simulink model "main_observer_sim1"  (R2015a)
settings: Solver=ode45  StartTime=0.0  StopTime=10  FixedStep=1e-4  MaxStep=1e-3  RelTol=1e-3
values from neighbouring files (symbols this model uses):
  A = sys_rand.A    [main_Observer_states.m]
  C = [0.617255113405149,0,0,-0.448535555941661,0.134230346538703,1.41932930409004;0.283640603624291,0,2.22808153625508,-1.86462753317668,-1.99763494036701,-0.0116516666362024;0.350975702033898,-0.174162030842294,1.44167650824058,-0.392420914284623,1.30288133017051,-0.392171726620127]    [finding_Y.m]    (also in main_Observer_states.m = sys_rand.C)
  Gama = eta*A-X*C    [main_Observer_states.m]    (also in observer.mat = [-0.665415381788 -1.71297839543 -11.0757301234 9.21615917151)
  H = B(:,end)    [main_Observer_states.m]
  Phi = dec2mat(LMISYS,xopt,2)    [main_Observer_states.m]    (also in observer.mat = [2.03974430811 -0.144807404976 -3.64797116197 7.53997403465 )
  theta = theta1+Y*theta2    [main_Observer_states.m]    (also in observer.mat = [-0.848682280391 0.936204937086 2.9983152382 2.21151006385 4)
settings Model: Creator=p4wp4w  LastModifiedBy=p4wp4w

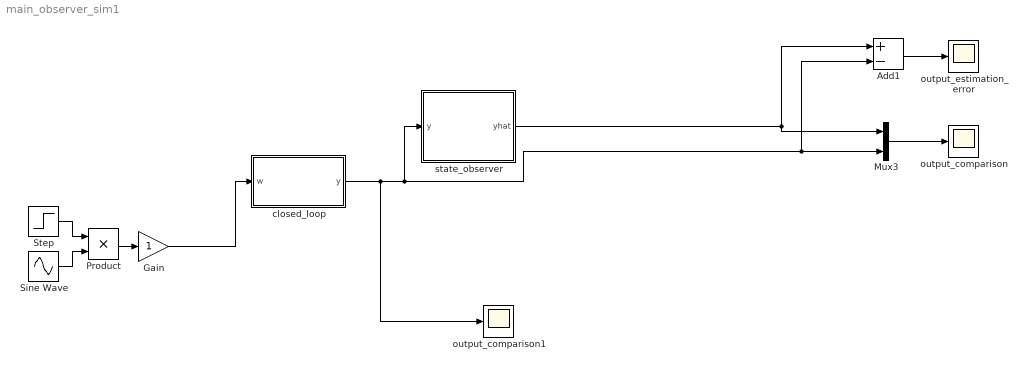
== system main_observer_sim1 ==
  Add1 : Sum  Inputs=+-
  Gain : Gain
  Mux3 : Mux  Inputs=2
  Product : Product
  Sine Wave : Sin  Frequency=10  SampleTime=0
  Step : Step  Before=8  After=0  SampleTime=0
  closed_loop : Subsystem
  output_comparison : Scope
      settings: YMin=-0.00125  YMax=0.003
  output_comparison1 : Scope
      settings: YMin=-0.0024  YMax=-2.1684e-19  SaveName=ScopeData5
  output_estimation_error : Scope
      settings: YMin=-0.0024  YMax=-2.1684e-19  SaveName=errorval
  state_observer : Subsystem
  wires:
  closed_loop/1(y) -> output_comparison1/1, Add1/2, Mux3/2, state_observer/1(y)
  Mux3/1 -> output_comparison/1
  state_observer/1(yhat) -> Mux3/1, Add1/1
  Gain/1 -> closed_loop/1(w)
  Add1/1 -> output_estimation_error/1
  Product/1 -> Gain/1
  Step/1 -> Product/1
  Sine Wave/1 -> Product/2

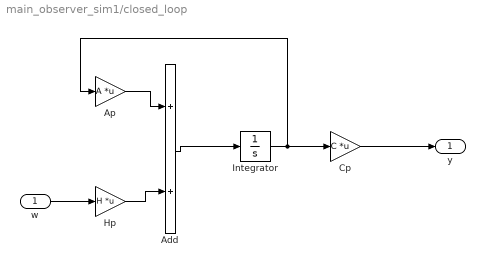
== system main_observer_sim1/closed_loop ==
  w : Inport
  Add : Sum
  Ap : Gain  Gain=A  Multiplication=Matrix(K*u)
  Cp : Gain  Gain=C  Multiplication=Matrix(K*u)
  Hp : Gain  Gain=H  Multiplication=Matrix(K*u)
  Integrator : Integrator
  y : Outport
  wires:
  w/1 -> Hp/1
  Add/1 -> Integrator/1
  Integrator/1 -> Cp/1, Ap/1
  Ap/1 -> Add/1
  Hp/1 -> Add/2
  Cp/1 -> y/1

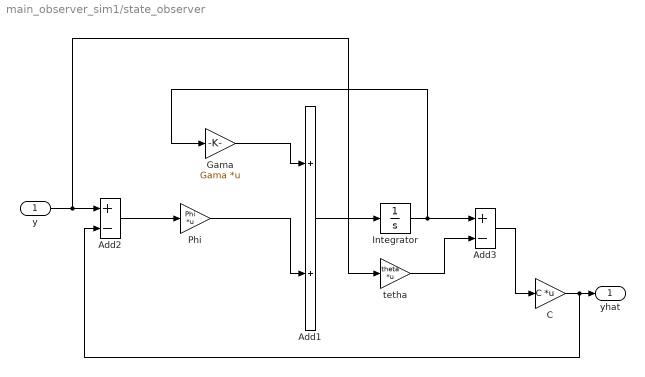
== system main_observer_sim1/state_observer ==
  y : Inport
  Add1 : Sum
  Add2 : Sum  Inputs=+-
  Add3 : Sum  Inputs=+-
  C : Gain  Gain=C  Multiplication=Matrix(K*u)
  Gama : Gain  Gain=Gama  Multiplication=Matrix(K*u)
  Integrator : Integrator
  Phi : Gain  Gain=Phi  Multiplication=Matrix(K*u)
  tetha : Gain  Gain=theta  Multiplication=Matrix(K*u)
  yhat : Outport
  wires:
  y/1 -> tetha/1, Add2/1
  C/1 -> Add2/2, yhat/1
  Add1/1 -> Integrator/1
  Gama/1 -> Add1/1
  Integrator/1 -> Gama/1, Add3/1
  Phi/1 -> Add1/2
  Add2/1 -> Phi/1
  tetha/1 -> Add3/2
  Add3/1 -> C/1
